simulink model "buzzer_module"  (R2021b)
settings: Solver=FixedStepAuto  StartTime=0.0  StopTime=inf  RelTol=1e-3
libraries: arduinolib x3, simulink x1, arduinosensorlib x1
settings Model: ExtModeTrigDuration=2  Creator=snowg  LastModifiedBy=snowg
settings OptimizationCC: EnhancedBackFolding=on  PassReuseOutputArgsAs=Individual arguments  ZeroExternalMemoryAtStartup=off  ZeroInternalMemoryAtStartup=off  MaxStackSize=64  OptimizeBlockOrder=speed  DifferentSizesBufferReuse=on  OptimizationCustomize=off  EfficientTunableParamExpr=on
settings DebuggingCC: ParameterTunabilityLossMsg=error
settings HardwareCC: ProdBitPerInt=16  ProdBitPerPointer=16  ProdBitPerSizeT=16  ProdBitPerPtrDiffT=16  ProdLargestAtomicFloat=None  ProdWordSize=8  ProdHWDeviceType=Atmel->AVR
settings SFSimCC: MATLABDynamicMemAlloc=off
settings RTWCC: Description=Embedded Coder  SystemTargetFile=ert.tlc  HardwareBoard=Arduino Mega 2560  TemplateMakefile=ert_default_tmf  Toolchain=Arduino AVR
settings CodeAppCC: ForceParamTrailComments=on  IgnoreCustomStorageClasses=off  OperatorAnnotations=on  SimulinkDataObjDesc=on  SFDataObjDesc=on  InsertBlockDesc=on
settings ERTTargetCC: SupportContinuousTime=on  SupportVariableSizeSignals=on  ExtModeTransport=3  ExtModeStaticAlloc=on  ExtModeStaticAllocSize=2048  ExtModeMexFile=ext_xcp  ExtModeIntrfLevel=Level2 - Open

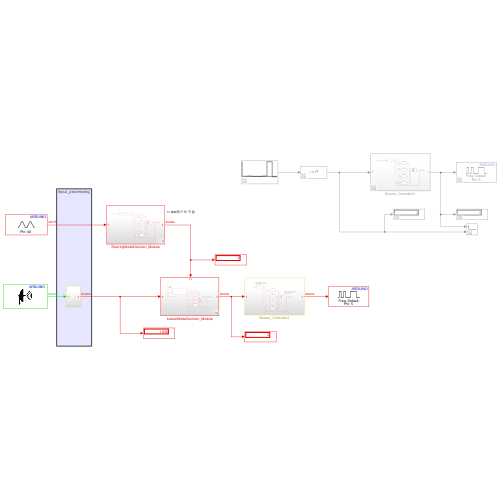
[thumbnail: Simulink's stored preview of the top-level diagram]
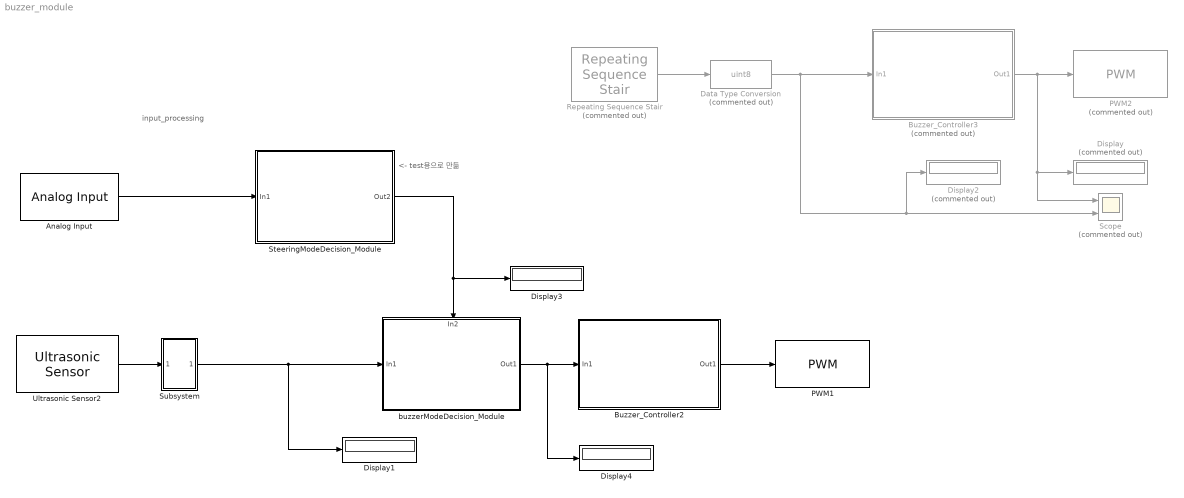
== system buzzer_module ==
  note: <- test용으로 만듦
  note: input_processing
  Analog Input : arduinolib/Analog Input  pinNumber=0  ReadResultsOnly=off  ConversionTriggerSource=Software  ExternalTriggerType=uint32( 0 )  OutputDataType=uint16  EnableConversionCompleteNotify=off  EnableOuputStatus=off  SampleTime=-1  blockPlatform=arduino
  Buzzer_Controller2 : Subsystem
  Buzzer_Controller3 : Subsystem  Commented=on
  Data Type Conversion : DataTypeConversion  Commented=on  OutDataTypeStr=uint8
  Display : Display  Commented=on
  Display1 : Display
  Display2 : Display  Commented=on
  Display3 : Display
  Display4 : Display
  PWM1 : arduinolib/PWM  pinNumber=5  frequencyType=Default  desiredFrequency=490.2  achievableFrequency=490.2
  PWM2 : arduinolib/PWM  Commented=on  pinNumber=5  frequencyType=Default  desiredFrequency=490.2  achievableFrequency=490.2
  Repeating Sequence Stair : simulink/Sources/Repeating Sequence Stair  Commented=on  OutValues=[0 2 0 1 3 100 -2].'  tsamp=2  OutMin=[]  OutMax=[]  OutDataTypeStr=double  OutputDataTypeScalingMode=double  OutDataType=fixdt(0,8)  ConRadixGroup=Best Precision: Vector-wise  OutScaling=2^-12
  Scope : Scope  Commented=on  NumInputPorts=2
  SteeringModeDecision_Module : Subsystem
  Subsystem : Subsystem
  Ultrasonic Sensor2 : arduinosensorlib/Ultrasonic Sensor  NumSignalPins=2  TrigPin=24  EchoPin=26  SignalPin=3  SampleTime_=0.1  blockPlatform=ARDUINO
      settings: SourceProductBaseCode=ARDUINO
  buzzerModeDecision_Module : Subsystem
      settings: PortSchema="{\"entries\":[{\"content\":{\"sides\":[{\"content\":{\"connectorIds\":[\"In1\"]},\"type\":\"ConnectorPlacement.EquallySpacedRectSide\",\"uuid\":\"3bfd8a6a-6750-43b9-a34d-1030ee4edf99\"},{\"content\":{\"connectorIds\":[\"Out1\"],\"side\":\"RIGHT\"},\"type\":\"ConnectorPlacement.EquallySpacedRectSide\",\"uuid\":\"183584f3-ff01-485d-aa62-5859e0907314\"},{\"content\":{\"connectorIds\":[\"In2\"],\"side\":\"TOP\"},\"type\":\"ConnectorPlacement.EquallySpacedRectSide\",\"uuid\":\"c1dfd82e-f053-4e34-bada-190db50d8d84\"}]},\"type\":\"ConnectorPlacement.EquallySpacedConnector\",\"uuid\":\"77a311fc-b440-4422-9bc9-ecab92f49ada\"}],\"packageUris\":[\"http://schema.mathworks.com/mf0/Connector/R2020b\"],\"version\":\"1.0\"}"
  wires:
  Buzzer_Controller3/1(Out1) -> Scope/1, Display/1, PWM2/1
  Analog Input/1 -> SteeringModeDecision_Module/1(In1)
  SteeringModeDecision_Module/1(Out2) -> Display3/1, buzzerModeDecision_Module/2(In2)
  Ultrasonic Sensor2/1 -> Subsystem/1(In1)
  Subsystem/1(Out1) -> Display1/1, buzzerModeDecision_Module/1(In1)
  Repeating Sequence Stair/1 -> Data Type Conversion/1
  Data Type Conversion/1 -> Buzzer_Controller3/1(In1), Scope/2, Display2/1
  buzzerModeDecision_Module/1(Out1) -> Display4/1, Buzzer_Controller2/1(In1)
  Buzzer_Controller2/1(Out1) -> PWM1/1

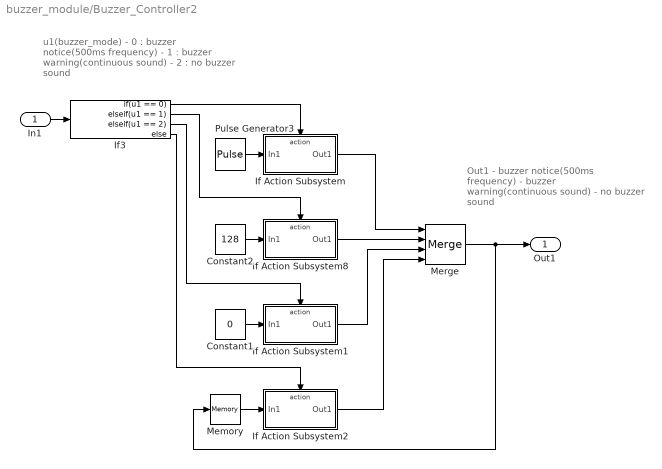
== system buzzer_module/Buzzer_Controller2 ==
  note: u1(buzzer_mode)
      | - 0 : buzzer notice(500ms frequency)
      | - 1 : buzzer warning(continuous sound)
      | - 2 : no buzzer sound
  note: Out1
      | - buzzer notice(500ms frequency)
      | - buzzer warning(continuous sound)
      | - no buzzer sound
  In1 : Inport
  Constant1 : Constant  Value=0
  Constant2 : Constant  Value=128  OutDataTypeStr=double
  If Action Subsystem : Subsystem  TreatAsAtomicUnit=on
  If Action Subsystem1 : Subsystem  TreatAsAtomicUnit=on
  If Action Subsystem2 : Subsystem  TreatAsAtomicUnit=on
  If Action Subsystem8 : Subsystem  TreatAsAtomicUnit=on
  If3 : If  IfExpression=u1 == 0  ElseIfExpressions=u1 == 1, u1 == 2
  Memory : Memory
  Merge : Merge  Inputs=4
  Pulse Generator3 : DiscretePulseGenerator  PulseType=Time based  Amplitude=128  Period=0.5  PulseWidth=50
  Out1 : Outport
  wires:
  Constant1/1 -> If Action Subsystem1/1(In1)
  If Action Subsystem1/1(Out1) -> Merge/3
  Pulse Generator3/1 -> If Action Subsystem/1(In1)
  Merge/1 -> Memory/1, Out1/1
  If3/2 -> If Action Subsystem8/Action
  Constant2/1 -> If Action Subsystem8/1(In1)
  If Action Subsystem/1(Out1) -> Merge/1
  In1/1 -> If3/1
  If3/1 -> If Action Subsystem/Action
  Memory/1 -> If Action Subsystem2/1(In1)
  If3/4 -> If Action Subsystem2/Action
  If3/3 -> If Action Subsystem1/Action
  If Action Subsystem2/1(Out1) -> Merge/4
  If Action Subsystem8/1(Out1) -> Merge/2

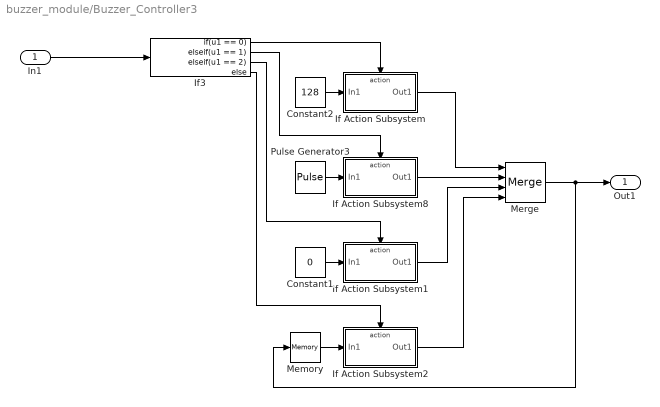
== system buzzer_module/Buzzer_Controller3 ==
  In1 : Inport
  Constant1 : Constant  Value=0
  Constant2 : Constant  Value=128  OutDataTypeStr=double
  If Action Subsystem : Subsystem  TreatAsAtomicUnit=on
  If Action Subsystem1 : Subsystem  TreatAsAtomicUnit=on
  If Action Subsystem2 : Subsystem  TreatAsAtomicUnit=on
  If Action Subsystem8 : Subsystem  TreatAsAtomicUnit=on
  If3 : If  IfExpression=u1 == 0  ElseIfExpressions=u1 == 1, u1 == 2
  Memory : Memory
  Merge : Merge  Inputs=4
  Pulse Generator3 : DiscretePulseGenerator  PulseType=Time based  Amplitude=5  Period=0.5  PulseWidth=50
  Out1 : Outport
  wires:
  Constant1/1 -> If Action Subsystem1/1(In1)
  If Action Subsystem1/1(Out1) -> Merge/3
  Constant2/1 -> If Action Subsystem/1(In1)
  Merge/1 -> Memory/1, Out1/1
  If3/2 -> If Action Subsystem8/Action
  Pulse Generator3/1 -> If Action Subsystem8/1(In1)
  If Action Subsystem/1(Out1) -> Merge/1
  In1/1 -> If3/1
  If3/1 -> If Action Subsystem/Action
  Memory/1 -> If Action Subsystem2/1(In1)
  If3/4 -> If Action Subsystem2/Action
  If3/3 -> If Action Subsystem1/Action
  If Action Subsystem2/1(Out1) -> Merge/4
  If Action Subsystem8/1(Out1) -> Merge/2

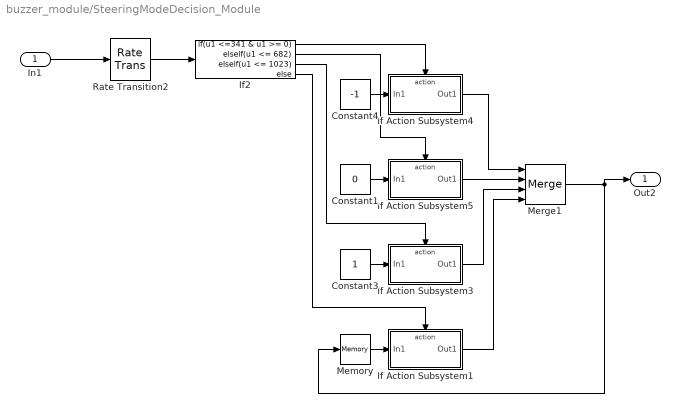
== system buzzer_module/SteeringModeDecision_Module ==
  In1 : Inport
  Constant1 : Constant  Value=0
  Constant3 : Constant
  Constant4 : Constant  Value=-1
  If Action Subsystem1 : Subsystem  TreatAsAtomicUnit=on
  If Action Subsystem3 : Subsystem  TreatAsAtomicUnit=on
  If Action Subsystem4 : Subsystem  TreatAsAtomicUnit=on
  If Action Subsystem5 : Subsystem  TreatAsAtomicUnit=on
  If2 : If  IfExpression=u1 <=341 & u1 >= 0  ElseIfExpressions=u1 <= 682, u1 <= 1023
  Memory : Memory
  Merge1 : Merge  Inputs=4
  Rate Transition2 : RateTransition  OutPortSampleTime=0.01
  Out2 : Outport
  wires:
  If Action Subsystem3/1(Out1) -> Merge1/3
  Constant3/1 -> If Action Subsystem3/1(In1)
  In1/1 -> Rate Transition2/1
  If2/2 -> If Action Subsystem5/Action
  Constant4/1 -> If Action Subsystem4/1(In1)
  If Action Subsystem5/1(Out1) -> Merge1/2
  If Action Subsystem4/1(Out1) -> Merge1/1
  Constant1/1 -> If Action Subsystem5/1(In1)
  If2/1 -> If Action Subsystem4/Action
  Rate Transition2/1 -> If2/1
  Merge1/1 -> Out2/1, Memory/1
  Memory/1 -> If Action Subsystem1/1(In1)
  If Action Subsystem1/1(Out1) -> Merge1/4
  If2/4 -> If Action Subsystem1/Action
  If2/3 -> If Action Subsystem3/Action

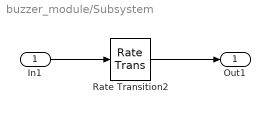
== system buzzer_module/Subsystem ==
  In1 : Inport
  Rate Transition2 : RateTransition  OutPortSampleTime=0.01
  Out1 : Outport
  wires:
  In1/1 -> Rate Transition2/1
  Rate Transition2/1 -> Out1/1

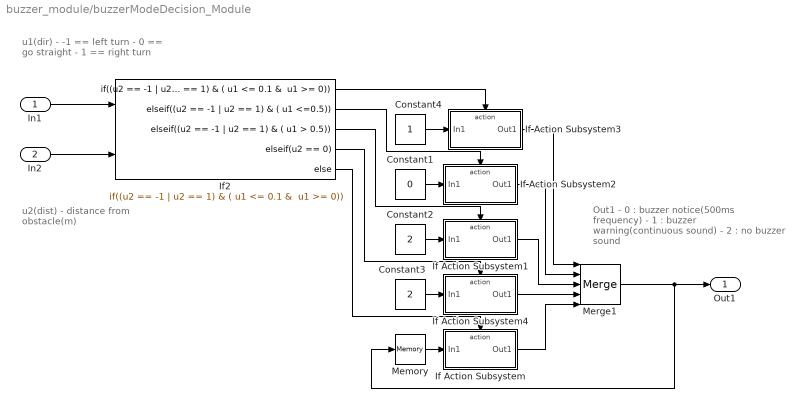
== system buzzer_module/buzzerModeDecision_Module ==
  note: u1(dir)
      | - -1 == left turn
      | - 0 == go straight
      | - 1 == right turn
  note: u2(dist)
      | - distance from obstacle(m)
  note: Out1
      | - 0 : buzzer notice(500ms frequency)
      | - 1 : buzzer warning(continuous sound)
      | - 2 : no buzzer sound
  In1 : Inport
  In2 : Inport  Port=2
  Constant1 : Constant  Value=0
  Constant2 : Constant  Value=2
  Constant3 : Constant  Value=2
  Constant4 : Constant
  If Action Subsystem : Subsystem  TreatAsAtomicUnit=on
  If Action Subsystem1 : Subsystem  TreatAsAtomicUnit=on
  If Action Subsystem2 : Subsystem  TreatAsAtomicUnit=on
  If Action Subsystem3 : Subsystem  TreatAsAtomicUnit=on
  If Action Subsystem4 : Subsystem  TreatAsAtomicUnit=on
  If2 : If  NumInputs=2  IfExpression="(u2 == -1 | u2 == 1) & ( u1 <= 0.1 &  u1 >= 0)"  ElseIfExpressions="(u2 == -1 | u2 == 1) & ( u1 <=0.5), (u2 == -1 | u2 == 1) & ( u1 > 0.5),  u2 == 0"
  Memory : Memory
  Merge1 : Merge  Inputs=5
  Out1 : Outport
  wires:
  If Action Subsystem/1(Out1) -> Merge1/5
  If2/5 -> If Action Subsystem/Action
  Memory/1 -> If Action Subsystem/1(In1)
  If2/2 -> If Action Subsystem2/Action
  Constant4/1 -> If Action Subsystem3/1(In1)
  If Action Subsystem2/1(Out1) -> Merge1/2
  If Action Subsystem3/1(Out1) -> Merge1/1
  Constant1/1 -> If Action Subsystem2/1(In1)
  If2/1 -> If Action Subsystem3/Action
  In1/1 -> If2/1
  Merge1/1 -> Out1/1, Memory/1
  In2/1 -> If2/2
  Constant2/1 -> If Action Subsystem1/1(In1)
  If Action Subsystem1/1(Out1) -> Merge1/3
  If2/4 -> If Action Subsystem4/Action
  If2/3 -> If Action Subsystem1/Action
  Constant3/1 -> If Action Subsystem4/1(In1)
  If Action Subsystem4/1(Out1) -> Merge1/4

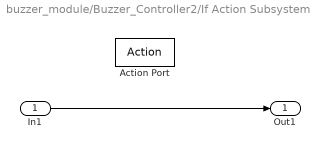
== system buzzer_module/Buzzer_Controller2/If Action Subsystem ==
  In1 : Inport
  Action Port : ActionPort  ActionPortLabel=if(u1 == 0)
  Out1 : Outport
  wires:
  In1/1 -> Out1/1

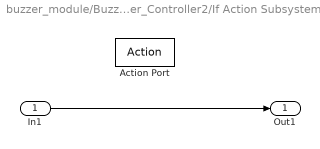
== system buzzer_module/Buzzer_Controller2/If Action Subsystem1 ==
  In1 : Inport
  Action Port : ActionPort  ActionPortLabel=elseif( u1 == 2)
  Out1 : Outport  LockScale=on
  wires:
  In1/1 -> Out1/1

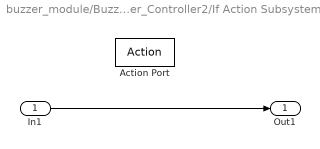
== system buzzer_module/Buzzer_Controller2/If Action Subsystem2 ==
  In1 : Inport
  Action Port : ActionPort  ActionPortLabel=else
  Out1 : Outport
  wires:
  In1/1 -> Out1/1

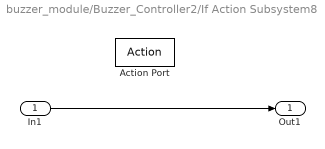
== system buzzer_module/Buzzer_Controller2/If Action Subsystem8 ==
  In1 : Inport
  Action Port : ActionPort  ActionPortLabel=elseif(u1 == 1)
  Out1 : Outport
  wires:
  In1/1 -> Out1/1

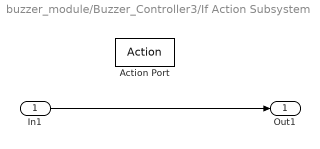
== system buzzer_module/Buzzer_Controller3/If Action Subsystem ==
  In1 : Inport
  Action Port : ActionPort  ActionPortLabel=if(u1 == 0)
  Out1 : Outport
  wires:
  In1/1 -> Out1/1

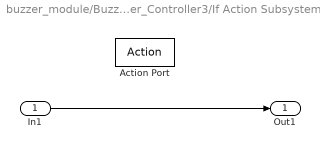
== system buzzer_module/Buzzer_Controller3/If Action Subsystem1 ==
  In1 : Inport
  Action Port : ActionPort  ActionPortLabel=elseif( u1 == 2)
  Out1 : Outport  LockScale=on
  wires:
  In1/1 -> Out1/1

== system buzzer_module/Buzzer_Controller3/If Action Subsystem2 ==
  In1 : Inport
  Action Port : ActionPort  ActionPortLabel=else
  Out1 : Outport
  wires:
  In1/1 -> Out1/1

== system buzzer_module/Buzzer_Controller3/If Action Subsystem8 ==
  In1 : Inport
  Action Port : ActionPort  ActionPortLabel=elseif(u1 == 1)
  Out1 : Outport
  wires:
  In1/1 -> Out1/1

== system buzzer_module/SteeringModeDecision_Module/If Action Subsystem1 ==
  In1 : Inport
  Action Port : ActionPort  ActionPortLabel=else
  Out1 : Outport
  wires:
  In1/1 -> Out1/1

== system buzzer_module/SteeringModeDecision_Module/If Action Subsystem3 ==
  In1 : Inport
  Action Port : ActionPort  ActionPortLabel=elseif( u1 <= 1023)
  Out1 : Outport
  wires:
  In1/1 -> Out1/1

== system buzzer_module/SteeringModeDecision_Module/If Action Subsystem4 ==
  In1 : Inport
  Action Port : ActionPort  ActionPortLabel=if(u1 <=341 & u1 >= 0)
  Out1 : Outport
  wires:
  In1/1 -> Out1/1

== system buzzer_module/SteeringModeDecision_Module/If Action Subsystem5 ==
  In1 : Inport
  Action Port : ActionPort  ActionPortLabel=elseif(u1 <= 682)
  Out1 : Outport
  wires:
  In1/1 -> Out1/1

== system buzzer_module/buzzerModeDecision_Module/If Action Subsystem ==
  In1 : Inport
  Action Port : ActionPort  ActionPortLabel=else
  Out1 : Outport
  wires:
  In1/1 -> Out1/1

== system buzzer_module/buzzerModeDecision_Module/If Action Subsystem1 ==
  In1 : Inport
  Action Port : ActionPort  ActionPortLabel=elseif( (u2 == -1 | u2 == 1) & ( u1 > 0.5))
  Out1 : Outport
  wires:
  In1/1 -> Out1/1

== system buzzer_module/buzzerModeDecision_Module/If Action Subsystem2 ==
  In1 : Inport
  Action Port : ActionPort  ActionPortLabel=elseif((u2 == -1 | u2 == 1) & ( u1 <=0.5))
  Out1 : Outport
  wires:
  In1/1 -> Out1/1

== system buzzer_module/buzzerModeDecision_Module/If Action Subsystem3 ==
  In1 : Inport
  Action Port : ActionPort  ActionPortLabel="if((u2 == -1 | u2 == 1) & ( u1 <= 0.1 &  u1 >= 0))"
  Out1 : Outport
  wires:
  In1/1 -> Out1/1

== system buzzer_module/buzzerModeDecision_Module/If Action Subsystem4 ==
  In1 : Inport
  Action Port : ActionPort  ActionPortLabel="elseif(  u2 == 0)"
  Out1 : Outport
  wires:
  In1/1 -> Out1/1
